simulink model "Sim2e"  (R2016a)
settings: Solver=VariableStepAuto  StartTime=0.0  StopTime=100.0  RelTol=1e-3
values from neighbouring files (symbols this model uses):
  alpha_phi1 = 2.87    [modelParms.m]
  alpha_phi2 = -0.65    [modelParms.m]
  dist = deg2rad(2)    [modelParms.m]
  g = 9.8    [modelParms.m]
  k_d_phi = (2*zeta_phi*omega_n_phi - alpha_phi1)/alpha_phi2    [modelParms.m]
  k_i_chi = omega_n_chi^2*V_g/g    [AllResults.m]    (also in modelParms.m = omega_n_chi*V_g/g)
  k_i_phi = 0    [modelParms.m]
  k_p_chi = 2*zeta_chi*omega_n_chi*V_g/g    [AllResults.m]    (also in modelParms.m)
  k_p_phi = delta_a_max/e_phi_max * sign(alpha_phi2)    [modelParms.m]
  V_g = 637    [modelParms.m]
settings Model: Creator=Alex  LastModifiedBy=Alex

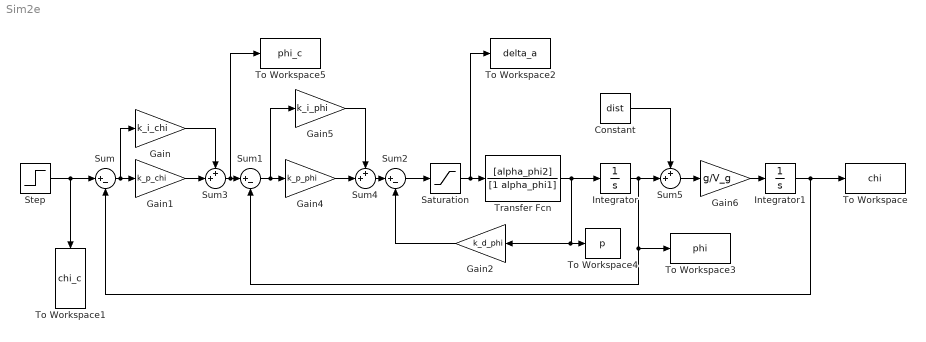
== system Sim2e ==
  Constant : Constant  Value=dist
  Gain : Gain  Gain=k_i_chi
  Gain1 : Gain  Gain=k_p_chi
  Gain2 : Gain  Gain=k_d_phi
  Gain4 : Gain  Gain=k_p_phi
  Gain5 : Gain  Gain=k_i_phi
  Gain6 : Gain  Gain=g/V_g
  Integrator : Integrator
  Integrator1 : Integrator
  Saturation : Saturate  UpperLimit=deg2rad(25)  LowerLimit=deg2rad(-25)
  Step : Step  After=deg2rad(5)  SampleTime=0
  Sum : Sum  Inputs=|+-
  Sum1 : Sum  Inputs=|+-
  Sum2 : Sum  Inputs=|+-
  Sum3 : Sum  Inputs=++|
  Sum4 : Sum  Inputs=++|
  Sum5 : Sum  Inputs=++|
  To Workspace : ToWorkspace  VariableName=chi  SaveFormat=Timeseries  SampleTime=-1
  To Workspace1 : ToWorkspace  VariableName=chi_c  SaveFormat=Timeseries  SampleTime=-1
  To Workspace2 : ToWorkspace  VariableName=delta_a  SaveFormat=Timeseries  SampleTime=-1
  To Workspace3 : ToWorkspace  VariableName=phi  SaveFormat=Timeseries  SampleTime=-1
  To Workspace4 : ToWorkspace  VariableName=p  SaveFormat=Timeseries  SampleTime=-1
  To Workspace5 : ToWorkspace  VariableName=phi_c  SaveFormat=Timeseries  SampleTime=-1
  Transfer Fcn : TransferFcn  Numerator=[alpha_phi2]  Denominator=[1 alpha_phi1]
  wires:
  Sum3/1 -> To Workspace5/1, Sum1/1
  Sum4/1 -> Sum2/1
  Sum/1 -> Gain/1, Gain1/1
  Gain1/1 -> Sum3/2
  Gain/1 -> Sum3/1
  Sum1/1 -> Gain5/1, Gain4/1
  Gain4/1 -> Sum4/2
  Gain5/1 -> Sum4/1
  Gain2/1 -> Sum2/2
  Gain6/1 -> Integrator1/1
  Sum5/1 -> Gain6/1
  Constant/1 -> Sum5/1
  Step/1 -> Sum/1, To Workspace1/1
  Transfer Fcn/1 -> Integrator/1, To Workspace4/1, Gain2/1
  Integrator/1 -> To Workspace3/1, Sum1/2, Sum5/2
  Integrator1/1 -> Sum/2, To Workspace/1
  Sum2/1 -> Saturation/1
  Saturation/1 -> To Workspace2/1, Transfer Fcn/1
